simulink model "Motor_Pos_cl"  (R2015a)
settings: Solver=ode15s  StartTime=0.0  StopTime=3  RelTol=1e-3
undefined symbols (not defined in the file or in its folder): b, J, K, kd, ki, kp, L, R, T0, T1
libraries: simulink x2
settings Model: Creator=maen  LastModifiedBy=Xiaotian
settings DataIOCC: SignalLoggingSaveFormat=ModelDataLogs
settings OptimizationCC: ExpressionDepthLimit=2147483647
settings DebuggingCC: UnderspecifiedInitializationDetection=Classic  MergeDetectMultiDrivingBlocksExec=none  FcnCallInpInsideContextMsg=UseLocalSettings  StateNameClashWarn=warning
settings GRTTargetCC: CombineOutputUpdateFcns=off  GRTInterface=on

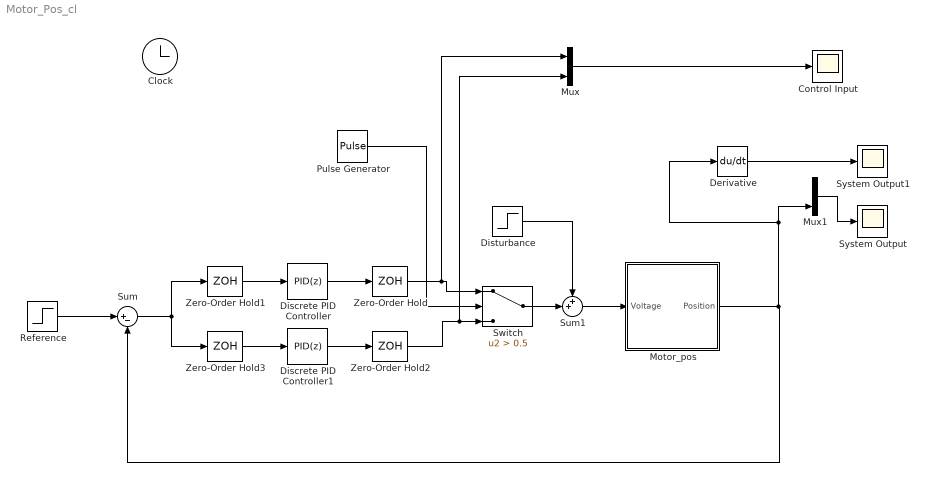
== system Motor_Pos_cl ==
  Clock : Clock
  Control Input : Scope
      settings: YMin=1.0025  YMax=1.04
  Derivative : Derivative
  Discrete PID Controller : simulink/Continuous/PID Controller  Controller=PID  TimeDomain=Discrete-time  SampleTime=T0  IntegratorMethod=Forward Euler  FilterMethod=Forward Euler  Form=Parallel  UseFilter=on  ControllerParametersSource=internal  P=kp  I=ki  D=kd  N=100  InitialConditionSource=internal  InitialConditionForIntegrator=0  InitialConditionForFilter=0  ExternalReset=none  LimitOutput=off  UpperSaturationLimit=inf  LowerSaturationLimit=-inf  LinearizeAsGain=off  AntiWindupMode=none  Kb=1  TrackingMode=off  Kt=1  PParamMin=[]  PParamMax=[]  IParamMin=[]  IParamMax=[]  DParamMin=[]  DParamMax=[]  NParamMin=[]  NParamMax=[]  KbParamMin=[]  KbParamMax=[]  KtParamMin=[]  KtParamMax=[]  POutMin=[]  POutMax=[]  IOutMin=[]  IOutMax=[]  DOutMin=[]  DOutMax=[]  NOutMin=[]  NOutMax=[]  KbOutMin=[]  KbOutMax=[]  KtOutMin=[]  KtOutMax=[]  IntegratorOutMin=[]  IntegratorOutMax=[]  FilterOutMin=[]  FilterOutMax=[]  SumOutMin=[]  SumOutMax=[]  SumI1OutMin=[]  SumI1OutMax=[]  SumI2OutMin=[]  SumI2OutMax=[]  SumI3OutMin=[]  SumI3OutMax=[]  SumDOutMin=[]  SumDOutMax=[]  SaturationOutMin=[]  SaturationOutMax=[]  IntegratorContinuousStateAttributes=''  IntegratorStateMustResolveToSignalObject=off  IntegratorRTWStateStorageClass=Auto  FilterContinuousStateAttributes=''  FilterStateMustResolveToSignalObject=off  FilterRTWStateStorageClass=Auto  DifferentiatorICPrevScaledInput=0  DifferentiatorOutMin=[]  DifferentiatorOutMax=[]
  Discrete PID Controller1 : simulink/Continuous/PID Controller  Controller=PID  TimeDomain=Discrete-time  SampleTime=T1  IntegratorMethod=Forward Euler  FilterMethod=Forward Euler  Form=Parallel  UseFilter=on  ControllerParametersSource=internal  P=kp  I=ki  D=kd  N=100  InitialConditionSource=internal  InitialConditionForIntegrator=0  InitialConditionForFilter=0  ExternalReset=none  LimitOutput=off  UpperSaturationLimit=inf  LowerSaturationLimit=-inf  LinearizeAsGain=off  AntiWindupMode=none  Kb=1  TrackingMode=off  Kt=1  PParamMin=[]  PParamMax=[]  IParamMin=[]  IParamMax=[]  DParamMin=[]  DParamMax=[]  NParamMin=[]  NParamMax=[]  KbParamMin=[]  KbParamMax=[]  KtParamMin=[]  KtParamMax=[]  POutMin=[]  POutMax=[]  IOutMin=[]  IOutMax=[]  DOutMin=[]  DOutMax=[]  NOutMin=[]  NOutMax=[]  KbOutMin=[]  KbOutMax=[]  KtOutMin=[]  KtOutMax=[]  IntegratorOutMin=[]  IntegratorOutMax=[]  FilterOutMin=[]  FilterOutMax=[]  SumOutMin=[]  SumOutMax=[]  SumI1OutMin=[]  SumI1OutMax=[]  SumI2OutMin=[]  SumI2OutMax=[]  SumI3OutMin=[]  SumI3OutMax=[]  SumDOutMin=[]  SumDOutMax=[]  SaturationOutMin=[]  SaturationOutMax=[]  IntegratorContinuousStateAttributes=''  IntegratorStateMustResolveToSignalObject=off  IntegratorRTWStateStorageClass=Auto  FilterContinuousStateAttributes=''  FilterStateMustResolveToSignalObject=off  FilterRTWStateStorageClass=Auto  DifferentiatorICPrevScaledInput=0  DifferentiatorOutMin=[]  DifferentiatorOutMax=[]
  Disturbance : Step  Time=0  After=0  SampleTime=0
  Motor_pos : Subsystem
  Mux : Mux  Inputs=2
  Mux1 : Mux  Inputs=2
  Pulse Generator : DiscretePulseGenerator  PulseType=Time based  Period=0.1  PulseWidth=10
  Reference : Step  Time=0  SampleTime=0
  Sum : Sum  Inputs=|+-
  Sum1 : Sum  Inputs=++|
  Switch : Switch  Criteria=u2 > Threshold  Threshold=0.5
  System Output : Scope
      settings: TimeRange=0.4130919490087732  YMin=0.9674716446821796  YMax=1.034963938230392
  System Output1 : Scope
      settings: YMin=1.0025  YMax=1.04  SaveName=ScopeData2
  Zero-Order Hold : ZeroOrderHold  SampleTime=T0
  Zero-Order Hold1 : ZeroOrderHold  SampleTime=T0
  Zero-Order Hold2 : ZeroOrderHold  SampleTime=T1
  Zero-Order Hold3 : ZeroOrderHold  SampleTime=T1
  wires:
  Motor_pos/1(Position) -> Sum/2, Mux1/2, Derivative/1
  Reference/1 -> Sum/1
  Sum1/1 -> Motor_pos/1(Voltage)
  Disturbance/1 -> Sum1/1
  Sum/1 -> Zero-Order Hold1/1, Zero-Order Hold3/1
  Switch/1 -> Sum1/2
  Zero-Order Hold1/1 -> Discrete PID Controller/1
  Discrete PID Controller/1 -> Zero-Order Hold/1
  Zero-Order Hold3/1 -> Discrete PID Controller1/1
  Discrete PID Controller1/1 -> Zero-Order Hold2/1
  Zero-Order Hold/1 -> Mux/1, Switch/1
  Zero-Order Hold2/1 -> Mux/2, Switch/3
  Mux/1 -> Control Input/1
  Pulse Generator/1 -> Switch/2
  Mux1/1 -> System Output/1
  Derivative/1 -> System Output1/1

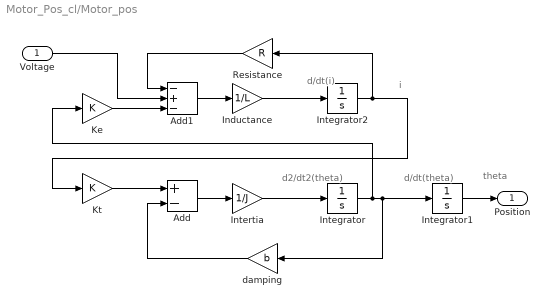
== system Motor_Pos_cl/Motor_pos ==
  note: i
  note: d/dt(theta)
  note: d2/dt2(theta)
  note: d/dt(i)
  note: theta
  Voltage : Inport
  Add : Sum  Inputs=+-
  Add1 : Sum  Inputs=-+-
  Inductance : Gain  Gain=1/L
  Integrator : Integrator
  Integrator1 : Integrator
  Integrator2 : Integrator
  Intertia : Gain  Gain=1/J
  Ke : Gain  Gain=K
  Kt : Gain  Gain=K
  Resistance : Gain  Gain=R
  damping : Gain  Gain=b
  Position : Outport
  wires:
  Inductance/1 -> Integrator2/1
  Integrator/1 -> Integrator1/1, damping/1, Ke/1
  Integrator1/1 -> Position/1
  Intertia/1 -> Integrator/1
  Integrator2/1 -> Kt/1, Resistance/1
  Add/1 -> Intertia/1
  Add1/1 -> Inductance/1
  Kt/1 -> Add/1
  damping/1 -> Add/2
  Ke/1 -> Add1/3
  Resistance/1 -> Add1/1
  Voltage/1 -> Add1/2
